simulink model "q3_TDO_v2"  (R2020b)
settings: Solver=ode4  StartTime=0.0  StopTime=SIM_TIME  FixedStep=STEP_SIZE  RelTol=1e-3
undefined symbols (not defined in the file): F_tf_d, T_s
libraries: cstblocks x8
settings Model: Creator=Theis  LastModifiedBy=Theis

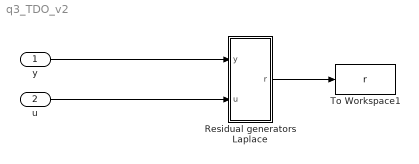
== system q3_TDO_v2 ==
  y : Inport
  u : Inport  Port=2
  Residual generators Laplace : Subsystem
  To Workspace1 : ToWorkspace  VariableName=r  SaveFormat=Timeseries  SampleTime=T_s
  wires:
  Residual generators Laplace/1(r) -> To Workspace1/1
  u/1 -> Residual generators Laplace/2(u)
  y/1 -> Residual generators Laplace/1(y)

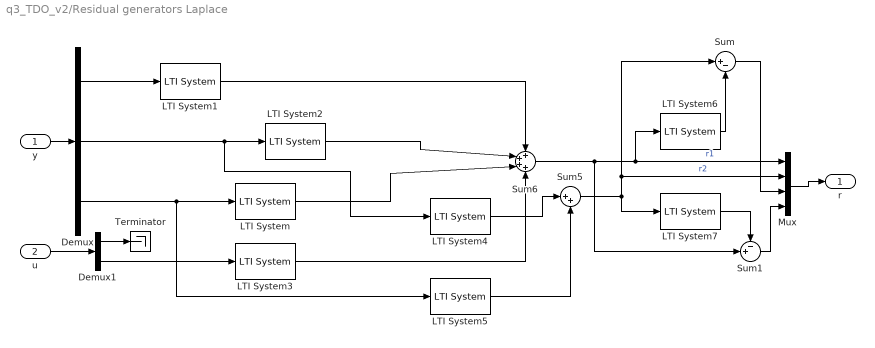
== system q3_TDO_v2/Residual generators Laplace ==
  y : Inport
  u : Inport  Port=2
  Demux : Demux  Outputs=3
  Demux1 : Demux  Outputs=2
  LTI System : cstblocks/LTI System  sys=F_tf_d(1,3)  IC=[]
  LTI System1 : cstblocks/LTI System  sys=F_tf_d(1,1)  IC=[]
  LTI System2 : cstblocks/LTI System  sys=F_tf_d(1,2)  IC=[]
  LTI System3 : cstblocks/LTI System  sys=F_tf_d(1,5)  IC=[]
  LTI System4 : cstblocks/LTI System  sys=F_tf_d(2,2)  IC=[]
  LTI System5 : cstblocks/LTI System  sys=F_tf_d(2,3)  IC=[]
  LTI System6 : cstblocks/LTI System  sys=r3_tf_d  IC=[]
  LTI System7 : cstblocks/LTI System  sys=r4_tf_d  IC=[]
  Mux : Mux
  Sum : Sum  Inputs=|+-
  Sum1 : Sum  Inputs=-+|
  Sum5 : Sum  Inputs=|++
  Sum6 : Sum  Inputs=++++
  Terminator : Terminator
  r : Outport  VectorParamsAs1DForOutWhenUnconnected=off
  wires:
  y/1 -> Demux/1
  Mux/1 -> r/1
  u/1 -> Demux1/1
  Demux1/1 -> Terminator/1
  Sum6/1 -> Sum1/2, LTI System6/1, Mux/1  "r1"
  Demux/1 -> LTI System1/1
  LTI System1/1 -> Sum6/1
  Demux/2 -> LTI System4/1, LTI System2/1
  LTI System2/1 -> Sum6/2
  Demux/3 -> LTI System5/1, LTI System/1
  LTI System/1 -> Sum6/3
  Demux1/2 -> LTI System3/1
  LTI System3/1 -> Sum6/4
  Sum5/1 -> Sum/1, Mux/2, LTI System7/1  "r2"
  LTI System4/1 -> Sum5/1
  LTI System5/1 -> Sum5/2
  LTI System6/1 -> Sum/2
  Sum/1 -> Mux/3
  Sum1/1 -> Mux/4
  LTI System7/1 -> Sum1/1
